simulink library "dspsnks4"  (Simulink 6.0)
settings: Solver=ode45  SolverMode=SingleTasking  StartTime=0.0  StopTime=10.0  RelTol=1e-3
undefined symbols (not defined in the file or in its folder): get, sdspwfall
libraries: dspspect3 x1, dspsigattribs x1, simulink x1
settings Model: RequirementInfo=9  CovMetricSettings=d  Creator=don  LastModifiedBy=mkhan  ExtModeAutoUpdateStatusClock=off
settings DataIOCC: SignalLoggingName=logsOut
settings OptimizationCC: BooleanDataType=off
settings DebuggingCC: CheckExecutionContextPreStartOutputMsg=on  CheckExecutionContextRuntimeOutputMsg=on  SolverPrmCheckMsg=none
settings HardwareCC: TargetUnknown=on
settings ModelReferenceCC: UpdateModelReferenceTargets=IfOutOfDate
settings GRTTargetCC: LifeSpan=inf
settings SFSimCC: SFSimApplyToAllLibs=on  SFSimBuildMode=Incremental

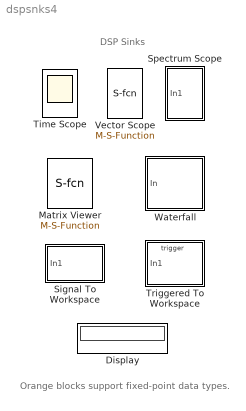
== system dspsnks4 ==
  note: DSP Sinks
  note: Orange blocks support fixed-point data types.
  Display : Display
      settings: CopyFcn=dspfixptcopycallback
  Matrix Viewer : M-S-Function  MFile=sdspmview2  mask(Matrix Viewer){ShowPortLabels=off, ImageParams=off, CMapStr=hot(256), YMin=-1.0, YMax=1.0, AxisColorbar=on, AxisParams=off, AxisOrigin=Upper left corner, XLabel=X-axis, YLabel=Y-axis, ZLabel=Z-axis, FigPos=get(0,'defaultfigureposition'), AxisZoom=off}
      mask prompts: ShowPortLabels "dummy"; ImageParams "-------------------------------- Show Image properties ------------------------------------"; CMapStr "Colormap matrix:"; YMin "Minimum input value:"; YMax "Maximum input value:"; AxisColorbar "Display colorbar"; AxisParams "-------------------------------- Show axis properties ----------------------------------------"; AxisOrigin "Axis origin:"; XLabel "X-axis title:"; YLabel "Y-axis title:"; ZLabel "Colorbar title:"; FigPos "Figure position:"; AxisZoom "Axis zoom"
      mask help: Display a matrix as an image, scaling the colormap to the specified input data range. Colormap must be an Nx3 matrix of RGB values. Type "help graph3d" at the MATLAB prompt for a list of predefined colormaps.
      mask init:
      | CMap = CMapStr;
      | s = dspblkmview2(ImageParams, CMap, YMin, YMax, AxisColorbar, AxisParams,  AxisOrigin, XLabel,  YLabel,  ZLabel, FigPos, AxisZoom);
      settings: NameChangeFcn=sdspmview2([],[],[],'BlockNameChange');  OpenFcn=dspblkDDOpen('MatrixViewer');
      settings: CopyFcn=|
      | sdspmview2([],[],[],'BlockCopy');
      | dspfixptcopycallback;
      settings: DeleteFcn=|
      | sdspmview2([],[],[],'BlockDelete');
      | dspblkDDClose;
      mask Help: web(dspbhelp);
      mask StyleString: checkbox,checkbox,edit,edit,edit,checkbox,checkbox,popup(Upper left corner|Lower left corner),edit,edit,edit,edit,checkbox
      mask Display: disp('Matrix\nViewer')
  Signal To Workspace : Subsystem  EnableExecutionContextPropagation=on  mask(Signal To Workspace){VariableName=yout, MaxDataPoints=inf, Decimation=1, FrameMode=Concatenate frames (2-D array), FixptAsFi=off}
      mask prompts: VariableName "Variable name:"; MaxDataPoints "Limit data points to last:"; FrameMode "Frames:"; FixptAsFi "Log fixed-point data as a fi object"
      mask help: Write input to specified array in MATLAB's main workspace. Data is not available until the simulation is stopped or paused.
      mask init:
      | ConcatFrames = dspblkstw2(FrameMode);
      settings: CopyFcn=|
      | dspfixptcopycallback;
      | dspblkcopystw(gcbh);
      mask Help: web(dspbhelp);
      mask StyleString: edit,edit,edit,popup(Concatenate frames (2-D array)|Log frames separately (3-D array)),checkbox
      mask Display: disp(VariableName)
  Spectrum Scope : Subsystem  TreatAsAtomicUnit=on  EnableExecutionContextPropagation=on  SimViewingDevice=on  mask(Spectrum Scope){ScopeProperties=on, Domain=Frequency, HorizSpan=1, UseBuffer=off, BufferSize=128, Overlap=64, inpFftLenInherit=off, FFTlength=128, numAvg=2, DisplayProperties=off, AxisGrid=on, Memory=off, FrameNumber=on, AxisLegend=off, AxisZoom=off, OpenScopeAtSimStart=on, OpenScopeImmediately=off, FigPos=get(0,'defaultfigureposition'), AxisProperties=off, XUnits=Hertz, XRange=[0...Fs/2], InheritXIncr=on, XIncr=1.0, XLabel=Samples, YUnits=dB, YMin=-10, YMax=10, YLabel=Magnitude, dB, LineProperties=off, LineDisables=, LineStyles=, LineMarkers=, LineColors=}
      mask prompts: ScopeProperties "-------------------------------- Show scope properties ------------------------------------"; Domain "Input domain:"; HorizSpan "Time display span (number of frames):"; UseBuffer "Buffer input"; BufferSize "Buffer size:"; Overlap "Buffer overlap:"; inpFftLenInherit "Specify FFT length"; FFTlength "FFT length:"; numAvg "Number of spectral averages:"; DisplayProperties "-------------------------------- Show display properties -----------------------------------"; AxisGrid "Show grid"; Memory "Persistence"; FrameNumber "Frame number"; AxisLegend "Channel legend"; AxisZoom "Compact display"; OpenScopeAtSimStart "Open scope at start of simulation"; OpenScopeImmediately "Open scope immediately"; FigPos "Scope position:"; AxisProperties "-------------------------------- Show axis properties ----------------------------------------"; XUnits "Frequency units:"; XRange "Frequency range:"; InheritXIncr "Inherit sample increment from input"; XIncr "Sample time of original time series:"; XLabel "X-axis title:"; YUnits "Amplitude scaling:"; YMin "Minimum Y-limit:"; YMax "Maximum Y-limit:"; YLabel "Y-axis title:"; LineProperties "-------------------------------- Show line properties -----------------------------------------"; LineDisables "Line visibility:"; LineStyles "Line styles:"; LineMarkers "Line markers:"; LineColors "Line colors:"
      mask help: Compute and display the periodogram of each input signal. Non-frame based inputs to the block should use the buffering option.
      mask init:
      | [x,y,str] = dspblkbfftscope2('icon');
      | s = dspblkbfftscope2('init');
      settings: NameChangeFcn=sdspfscope2([],[],[],'NameChange');  OpenFcn=dspblkDDOpen('SpectrumScope');  RTWSystemCode=Function
      settings: CopyFcn=|
      | sdspfscope2([],[],[],'BlockCopy');
      | dspfixptcopycallback
      settings: DeleteFcn=|
      | sdspfscope2([],[],[],'BlockDelete');
      | dspblkDDClose;
      mask Help: web(dspbhelp);
      mask StyleString: checkbox,popup(Time|Frequency|User-defined),edit,checkbox,edit,edit,checkbox,edit,edit,checkbox,checkbox,checkbox,checkbox,checkbox,checkbox,checkbox,checkbox,edit,checkbox,popup(Hertz|rad/sec),popup([0...Fs/2]|[-Fs/2...Fs/2]|[0...Fs]),checkbox,edit,edit,popup(Magnitude|dB),edit,edit,edit,checkbox,edit,edit,edit,edit
      mask CallbackString: dspblkbfftscope2('dynamic','ScopeProperties')|||dspblkbfftscope2('dynamic','useBuffer');|||dspblkbfftscope2('dynamic','FftLenCheckbox');|||dspblkbfftscope2('dynamic','DisplayProperties');|||||||dspblkbfftscope2('dynamic','OpenScope');||dspblkbfftscope2('dynamic','AxisProperties');|||dspblkbfftscope2('dynamic','InheritXIncr');|||||||dspblkbfftscope2('dynamic','LineProperties');||||
      mask Display: plot(x,y); text(14,20,str);
  Time Scope : Scope
      settings: CopyFcn=dspfixptcopycallback  DataFormat=Structure
  Triggered To Workspace : Subsystem  TreatAsAtomicUnit=on  EnableExecutionContextPropagation=on  mask(Triggered To Workspace){TriggerType=Rising edge, VariableName=yout, Buffer=1000, Decimation=1, FixptAsFi=off}
      mask prompts: TriggerType "Trigger type:"; VariableName "Variable name:"; Buffer "Maximum number of rows:"; FixptAsFi "Log fixed-point data as a fi object"
      mask help: Write input to specified variable in the workspace when trigger is received.
      mask init:
      | dspblktrigtwks('init',TriggerType);
      settings: CopyFcn=|
      | dspfixptcopycallback
      | dspblkcopystw(gcbh);
      mask Help: web(dspbhelp);
      mask StyleString: popup(Rising edge|Falling edge|Either edge),edit,edit,edit,checkbox
      mask Display: disp(VariableName);
  Vector Scope : M-S-Function  MFile=sdspfscope2  Parameters=1  mask(Vector Scope){ScopeProperties=on, Domain=Time, HorizSpan=1, DisplayProperties=off, AxisGrid=on, Memory=off, FrameNumber=on, AxisLegend=off, AxisZoom=off, OpenScopeAtSimStart=on, OpenScopeImmediately=off, FigPos=get(0,'defaultfigureposition'), AxisProperties=off, XUnits=Hertz, XRange=[0...Fs/2], InheritXIncr=on, XIncr=1, XLabel=Time, YUnits=dB, YMin=-10, YMax=10, YLabel=Amplitude, LineProperties=off, LineDisables=, LineStyles=, LineMarkers=, LineColors=, ShowPortLabels=off}
      mask prompts: ScopeProperties "-------------------------------- Show scope properties ------------------------------------"; Domain "Input domain:"; HorizSpan "Time display span (number of frames):"; DisplayProperties "-------------------------------- Show display properties -----------------------------------"; AxisGrid "Show grid"; Memory "Persistence"; FrameNumber "Frame number"; AxisLegend "Channel legend"; AxisZoom "Compact display"; OpenScopeAtSimStart "Open scope at start of simulation"; OpenScopeImmediately "Open scope immediately"; FigPos "Scope position:"; AxisProperties "-------------------------------- Show axis properties ----------------------------------------"; XUnits "Frequency units:"; XRange "Frequency range:"; InheritXIncr "Inherit sample increment from input"; XIncr "Increment per sample in input frame:"; XLabel "X-axis title:"; YUnits "Amplitude scaling:"; YMin "Minimum Y-limit:"; YMax "Maximum Y-limit:"; YLabel "Y-axis title:"; LineProperties "-------------------------------- Show line properties -----------------------------------------"; LineDisables "Line visibilities:"; LineStyles "Line styles:"; LineMarkers "Line markers:"; LineColors "Line colors:"; ShowPortLabels "dummy"
      mask help:
      | Display a vector or matrix of time-domain, frequency-domain, or user-specified data.  Each column of a 2-D input matrix is plotted as a separate data channel.  1-D inputs are assumed to be a single data channel.
      |
      | For frequency-domain operation, input should come from a source such as the Magnitude FFT block, or a block with equivalent data organization.
      mask init:
      | [x,y,str] = dspblkfscope2('icon');
      | s = dspblkfscope2('init');
      settings: NameChangeFcn=sdspfscope2([],[],[],'NameChange');  OpenFcn=dspblkDDOpen('VectorScope');
      settings: CopyFcn=|
      | sdspfscope2([],[],[],'BlockCopy');
      | dspfixptcopycallback
      settings: DeleteFcn=|
      | sdspfscope2([],[],[],'BlockDelete');
      | dspblkDDClose;
      mask Help: web(dspbhelp);
      mask StyleString: checkbox,popup(Time|Frequency|User-defined),edit,checkbox,checkbox,checkbox,checkbox,checkbox,checkbox,checkbox,checkbox,edit,checkbox,popup(Hertz|rad/sec),popup([0...Fs/2]|[-Fs/2...Fs/2]|[0...Fs]),checkbox,edit,edit,popup(Magnitude|dB),edit,edit,edit,checkbox,edit,edit,edit,edit,checkbox
      mask Display: plot(x,y); text(14,20,str);
  Waterfall : Subsystem  LoadFcn=sdspwfall([],[],[],'BlockLoad');  TreatAsAtomicUnit=on  EnableExecutionContextPropagation=on  SimViewingDevice=on  mask(Waterfall){TraceProperties=off, NumTraces=6, CMapStr=autumn, TNewest=1, TOldest=0, HistoryLength=10, HistoryFull=Overwrite, UpdateInterval=1, ExportMode=Selected, MLExportName=ExportData, AutoExport=off, DisplayProperties=off, MouseMode=Orbit, AxisGrid=on, Snapshot=off, Suspend=off, SyncSnapshots=off, OpenScopeAtSimStart=on, FigPos=[243 195 405 320], CameraView=[69.4600750684385 564.426060114276 -133.474523953492 0 18.5 3.5 0.616338299486424 -7.9078811427274 1.98411164834144 2.40985953613679 1 18.5 3], InportDimsHint=[32 1], AxisProperties=off, YMin=-1, YMax=1, AxisColor='w', XLabel=Amplitude, YLabel=Samples, ZLabel=Time, TriggerProperties=off, TrigStartMode=Immediately, TrigStartT=0, TrigStartN=0, TrigStartFcn=trigbegin, TrigStopMode=Never, TrigStopT=0.1, TrigStopN=1, TrigStopFcn=trigend, TrigRearmMode=Never, TrigRearmT=0, TrigRearmN=0, TrigRearmFcn=trigrearm, XformProperties=on, XformMode=None, XformFcn=abs, XformExpr=(u+1)/2}
      mask prompts: TraceProperties "-------------------------------- Show waterfall properties ------------------------------------"; NumTraces "Number of traces:"; CMapStr "Colormap name (jet, hot, etc):"; TNewest "Transparency of newest trace, 0 to 1 (1=opaque):"; TOldest "Transparency of oldest trace, 0 to 1:"; HistoryLength "History length:"; HistoryFull "History full:"; UpdateInterval "Display update interval:"; ExportMode "Data logging:"; MLExportName "MATLAB export variable name:"; AutoExport "Automatic export to workspace"; DisplayProperties "-------------------------------- Show display properties ----------------------------------------"; MouseMode "Mouse mode:"; AxisGrid "Show grid"; Snapshot "Snapshot (pause) display"; Suspend "Suspend data capture"; SyncSnapshots "Synchronize suspend/snapshot"; OpenScopeAtSimStart "Open scope at start of simulation"; FigPos "Scope position:"; CameraView "Camera view:"; InportDimsHint "Inport dimensions hint:"; AxisProperties "-------------------------------- Show axis properties ----------------------------------------"; YMin "Minimum input value:"; YMax "Maximum input value:"; AxisColor "Axis color:"; XLabel "X-axis title:"; YLabel "Y-axis title:"; ZLabel "Z-axis title:"; TriggerProperties "-------------------------------- Show trigger properties ----------------------------------------"; TrigStartMode "Begin recording:"; TrigStartT "Begin record time, T:"; TrigStartN "Begin record count, N:"; TrigStartFcn "Begin record function:"; TrigStopMode "Record until:"; TrigStopT "End record time, T:"; TrigStopN "End record count, N:"; TrigStopFcn "End record function:"; TrigRearmMode "Re-enable recording:"; TrigRearmT "Re-enable time, T:"; TrigRearmN "Re-enable count, N:"; TrigRearmFcn "Re-enable function:"; XformProperties "-------------------------------- Show transform properties ----------------------------------------"; XformMode "Transform:"; XformFcn "Function:"; XformExpr "Expression:"
      mask help:
      | Display sequence of vectors as a 3-D waterfall plot.  Input must be real-valued.  For matrix inputs, each column of data is treated as a sequential vector input to the waterfall.
      |
      | Colormap must be the name of a MATLAB colormap function, without arguments or parentheses.  Type "help graph3d" at the MATLAB prompt for a list of predefined colormaps.
      mask init:
      | if strcmp(Suspend,'on'),
      | 	str='Suspend';
      | elseif strcmp(Snapshot,'on'),
      | 	str='SnapShot';
      | else
      | 	str='';
      | end
      | sdspwfall([],[],[],'DialogApply');
      settings: DeleteFcn=sdspwfall([],[],[],'BlockDelete');  UndoDeleteFcn=sdspwfall([],[],[],'BlockUndoDelete');  NameChangeFcn=sdspwfall([],[],[],'BlockNameChange');  OpenFcn=sdspwfall([],[],[],'BlockOpen');  ErrorFcn=sdspwfall  RTWSystemCode=Function
      settings: CopyFcn=|
      | sdspwfall([],[],[],'BlockCopy');
      | dspfixptcopycallback
      mask Help: web(dspbhelp);
      mask StyleString: checkbox,edit,edit,edit,edit,edit,popup(Overwrite|Suspend|Extend),edit,popup(Selected|All visible|All history),edit,checkbox,checkbox,popup(Arrow|Orbit|Zoom),checkbox,checkbox,checkbox,checkbox,checkbox,edit,edit,edit,checkbox,edit,edit,edit,edit,edit,edit,checkbox,popup(Immediately|After T seconds|After N inputs|User-defined),edit,edit,edit,popup(Never|After T seconds|After N inputs|User-defined),edit,edit,edit,popup(Never|After T seconds|After N inputs|User-defined),edit,edit,edit,checkbox,popup(None|Amplitude->dB|Complex->Mag Lin|Complex->Mag dB|Complex->Angle|FFT->Mag Lin Fs/2|FFT->Mag dB Fs/2|FFT->Angle Fs/2|Power->dB|User-defined fcn|User-defined expr),edit,edit
      mask CallbackString: dspblkwfall('dynamic','TraceProperties');|||||||||||dspblkwfall('dynamic','DisplayProperties');||||||||||dspblkwfall('dynamic','AxisProperties');|||||||dspblkwfall('dynamic','TriggerProperties');|||||||||||||dspblkwfall('dynamic','XformProperties');|||
      mask Display:
      | disp('Waterfall\nScope\n')
      | color('red')
      | text(.08,.2,str)

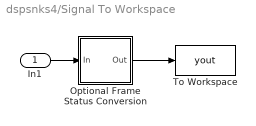
== system dspsnks4/Signal To Workspace ==
  In1 : Inport  LatchInput=off
  Optional Frame Status Conversion : Subsystem  EnableExecutionContextPropagation=on  mask(Replaceable Contents){oname=Frame Status, osrc=dspsigattribs/Frame Status Conversion, oargs={'outframe','Sample-based','growRefPort','off'}, replace=ConcatFrames}
      mask prompts: oname "Relative name of blocks to replace:"; osrc "Simulink path to each source block:"; oargs "Parameter/value pairs to each block:"; replace "Replace with short-circuit:"
      mask help: Configurable subsystem holding blocks which may be replaced by virtual short-circuits (muxes) when not needed.
      mask init:
      | opts.name = oname; opts.src = osrc; opts.args = oargs;
      | dspskipblk(gcb,opts,replace);
  To Workspace : ToWorkspace  VariableName=yout  SampleTime=-1  SaveFormat=Array
      settings: MaxDataPoints=MaxDataPoints  Decimation=Decimation
  wires:
  In1/1 -> Optional Frame Status Conversion/1(In)
  Optional Frame Status Conversion/1(Out) -> To Workspace/1

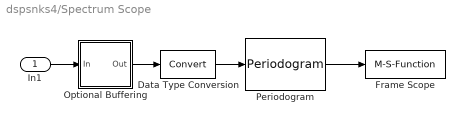
== system dspsnks4/Spectrum Scope ==
  In1 : Inport  LatchInput=off
  Data Type Conversion : DataTypeConversion  OutDataTypeMode=double  SaturateOnIntegerOverflow=on  RndMeth=Zero
  Frame Scope : M-S-Function  MFile=sdspfscope2  Parameters=2
      settings: CopyFcn=;
      mask Type: Frame Scope
      mask Description: Level-2 M-file S-function for frame scope.
      mask Help: web(dspbhelp);
      mask Display: disp('Frame\nScope')
  Optional Buffering : Subsystem  EnableExecutionContextPropagation=on  mask(Replaceable Contents){oname=Buffer, osrc=dspbuff3/Buffer, oargs={'N','BufferSize','V','Overlap','ic','0'}, replace=strcmp(UseBuffer,'off')}
      mask prompts: oname "Relative name of blocks to replace:"; osrc "Simulink path to each source block:"; oargs "Parameter/value pairs to each block:"; replace "Replace with short-circuit:"
      mask help: Configurable subsystem holding blocks which may be replaced by virtual short-circuits (muxes) when not needed.
      mask init:
      | opts.name = oname; opts.src = osrc; opts.args = oargs;
      | dspskipblk(gcb,opts,replace);
  Periodogram : dspspect3/Periodogram  wintype=Hann  Rs=50  beta=5  winsamp=Periodic  inheritFFT=on  fftsize=FFTlength  navg=numAvg
  wires:
  Data Type Conversion/1 -> Periodogram/1
  Optional Buffering/1(Out) -> Data Type Conversion/1
  In1/1 -> Optional Buffering/1(In)
  Periodogram/1 -> Frame Scope/1

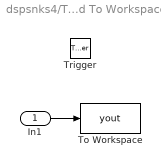
== system dspsnks4/Triggered To Workspace ==
  In1 : Inport  LatchInput=off
  Trigger : TriggerPort
  To Workspace : ToWorkspace  VariableName=yout  SampleTime=-1  SaveFormat=Array
      settings: MaxDataPoints=Buffer  Decimation=Decimation
  wires:
  In1/1 -> To Workspace/1

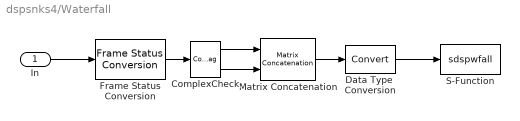
== system dspsnks4/Waterfall ==
  In : Inport  LatchInput=off
  ComplexCheck : ComplexToRealImag
  Data Type  Conversion : DataTypeConversion  OutDataTypeMode=double  SaturateOnIntegerOverflow=on  RndMeth=Zero
  Frame Status Conversion : dspsigattribs/Frame Status Conversion  growRefPort=off  outframe=Sample-based
  Matrix Concatenation : simulink/Math Operations/Matrix Concatenation  numInports=2  catMethod=Vertical
  S-Function : S-Function  FunctionName=sdspwfall
  wires:
  Data Type  Conversion/1 -> S-Function/1
  Matrix Concatenation/1 -> Data Type  Conversion/1
  ComplexCheck/2 -> Matrix Concatenation/2
  ComplexCheck/1 -> Matrix Concatenation/1
  In/1 -> Frame Status Conversion/1
  Frame Status Conversion/1 -> ComplexCheck/1

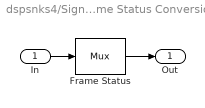
== system dspsnks4/Signal To Workspace/Optional Frame Status Conversion ==
  In : Inport  LatchInput=off
  Frame Status : Mux  Inputs=1
  Out : Outport  InitialOutput=0
  wires:
  Frame Status/1 -> Out/1
  In/1 -> Frame Status/1

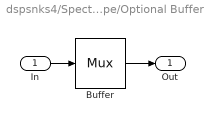
== system dspsnks4/Spectrum Scope/Optional Buffering ==
  In : Inport  LatchInput=off
  Buffer : Mux  Inputs=1
  Out : Outport  InitialOutput=0
  wires:
  In/1 -> Buffer/1
  Buffer/1 -> Out/1
